simulink model "doublMassControl"  (R2016b)
settings: Solver=VariableStepAuto  StartTime=0.0  StopTime=0.4  FixedStep=2e-4  RelTol=1e-3
values from neighbouring files (symbols this model uses):
  denGp = [m1*m2 0 (m1+m2)*k 0 0]    [doubleMassInit.m]
  denominator = denominator{1}    [doubleMassInit.m]    (also in mainFeedbackTuning.m)
  denQ = [1 2*wq*0.707 wq*wq]    [doubleMassInit.m]
  fs = 5000*2    (= 10000)    [doubleMassInit.m]    (also in mainFeedbackTuning.m)
  k = wn*wn*m1*m2/(m1+m2)    (= 25266187.2668)    [doubleMassInit.m]
  m11 = m1-1    (= 19)    [doubleMassInit.m]
  m22 = m2-0.5    (= 4.5)    [doubleMassInit.m]
  numerator = numerator{1}    [doubleMassInit.m]    (also in mainFeedbackTuning.m)
  numGp = k    (= 25266187.2668)    [doubleMassInit.m]
  numQ = wq*wq    (= 1421223033.76)    [doubleMassInit.m]
  Ts = 1/fs    (= 0.0001)    [doubleMassInit.m]    (also in mainFeedbackTuning.m)
libraries: simulink x6, model_controller x1
settings Model: Creator=Dai Luyao  LastModifiedBy=Dai Luyao

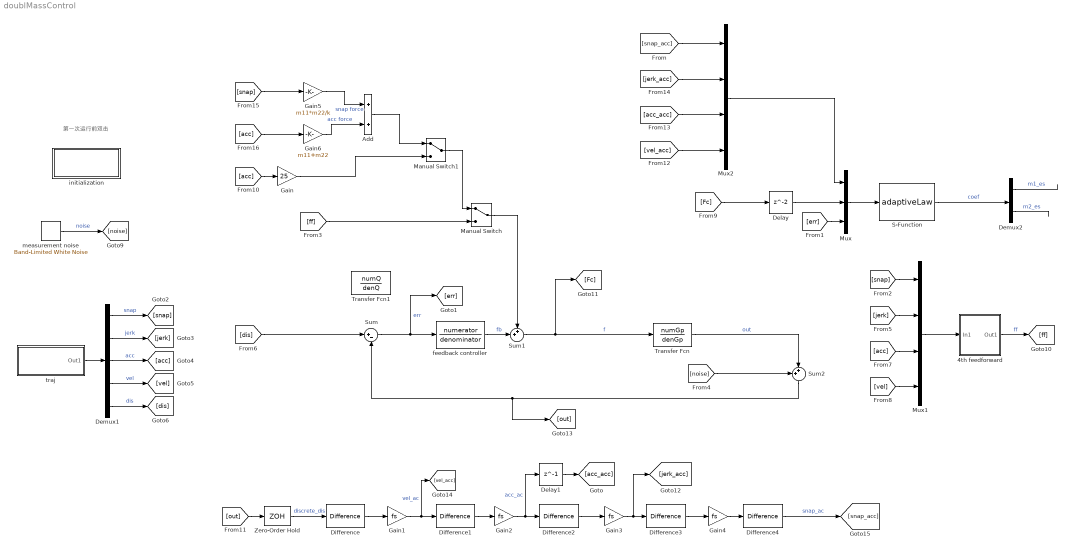
== system doublMassControl ==
  note: 第一次运行前双击
  4th feedforward : Subsystem
  Add : Sum
  Delay : Delay
  Delay1 : Delay  DelayLength=1
  Demux1 : Demux  Outputs=5
  Demux2 : Demux  Outputs=2
  Difference{,1..4} (5 alike) : simulink/Discrete/Difference  ICPrevInput=0.0  OutMin=[]  OutMax=[]  OutDataType=fixdt(1, 16)  OutScaling=2^-10  DoSatur=off
  Gain : Gain  Gain=25
  Gain{1..4} (4 alike) : Gain  Gain=fs
  Gain5 : Gain  Gain=m11*m22/k
  Gain6 : Gain  Gain=m11+m22
  Manual Switch : ManualSwitch
  Manual Switch1 : ManualSwitch
  Mux : Mux  Inputs=3
  Mux1 : Mux
  Mux2 : Mux
  S-Function : S-Function  FunctionName=adaptiveLaw  Parameters=1  SFunctionDeploymentMode=off  EnableBusSupport=off
  Sum : Sum  Inputs=|+-
  Sum1 : Sum  Inputs=++|
  Sum2 : Sum  Inputs=++|
  Transfer Fcn : TransferFcn  Numerator=numGp  Denominator=denGp
  Transfer Fcn1 : TransferFcn  Numerator=numQ  Denominator=denQ
  Zero-Order Hold : ZeroOrderHold  SampleTime=Ts
  feedback controller : TransferFcn  Numerator=numerator  Denominator=denominator
  initialization : Subsystem
      settings: OpenFcn=doubleMassInit;  MoveFcn=edit doubleMassInit;
  measurement noise : simulink/Sources/Band-Limited White Noise  Cov=noisePower  Ts=Ts  seed=[23341]
  traj : Subsystem  BlockChoice=4th order traj
      settings: AttributesFormatString=%<BlockChoice>  TemplateBlock=model_controller/Profile Generators/traj  MemberBlocks=2th order traj,3rd order traj,4th order traj,step
  wires:
  Sum/1 -> feedback controller/1, [err]  "err"
  feedback controller/1 -> Sum1/2  "fb"
  Sum1/1 -> Transfer Fcn/1, [Fc]  "f"
  Difference1/1 -> Gain2/1
  Difference/1 -> Gain1/1
  Gain1/1 -> [vel_acc], Difference1/1  "vel_ac"
  Mux/1 -> S-Function/1
  S-Function/1 -> Demux2/1  "coef"
  Zero-Order Hold/1 -> Difference/1  "discrete_dis"
  [err] -> Mux/3
  Delay/1 -> Mux/2
  Mux1/1 -> 4th feedforward/1(In1)
  measurement noise/1 -> [noise]  "noise"
  Transfer Fcn/1 -> Sum2/2  "out"
  [noise] -> Sum2/1
  Sum2/1 -> [out], Sum/2
  Demux1/1 -> [snap]  "snap"
  Demux1/2 -> [jerk]  "jerk"
  Demux1/3 -> [acc]  "acc"
  Demux1/4 -> [vel]  "vel"
  Demux1/5 -> [dis]  "dis"
  traj/1(Out1) -> Demux1/1
  [vel] -> Mux1/4
  [acc] -> Mux1/3
  [jerk] -> Mux1/2
  [snap] -> Mux1/1
  4th feedforward/1(Out1) -> [ff]  "ff"
  [Fc] -> Delay/1
  Difference2/1 -> Gain3/1
  Gain2/1 -> Delay1/1, Difference2/1  "acc_ac"
  Gain3/1 -> [jerk_acc], Difference3/1
  Gain4/1 -> Difference4/1
  Difference3/1 -> Gain4/1
  [out] -> Zero-Order Hold/1
  Difference4/1 -> [snap_acc]  "snap_ac"
  [snap_acc] -> Mux2/1
  [jerk_acc] -> Mux2/2
  [acc_acc] -> Mux2/3
  [vel_acc] -> Mux2/4
  Mux2/1 -> Mux/1
  Delay1/1 -> [acc_acc]
  Demux2/1 -> ?  "m1_es"
  Demux2/2 -> ?  "m2_es"
  [acc] -> Gain/1
  [snap] -> Gain5/1
  [acc] -> Gain6/1
  Gain5/1 -> Add/1  "snap force"
  Gain6/1 -> Add/2  "acc force"
  Add/1 -> Manual Switch1/1
  Gain/1 -> Manual Switch1/2
  Manual Switch1/1 -> Manual Switch/1
  [dis] -> Sum/1
  [ff] -> Manual Switch/2
  Manual Switch/1 -> Sum1/1

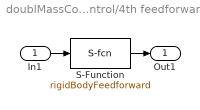
== system doublMassControl/4th feedforward ==
  In1 : Inport
  S-Function : S-Function  FunctionName=rigidBodyFeedforward  SFunctionDeploymentMode=off  EnableBusSupport=off
  Out1 : Outport
  wires:
  In1/1 -> S-Function/1
  S-Function/1 -> Out1/1

== system doublMassControl/initialization ==

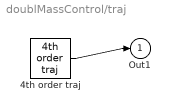
== system doublMassControl/traj ==
  4th order traj : model_controller/Profile Generators/4th order traj  t0=0  x=0.06  v=0.25  a=10  j=800  d=64000  Ts=0
  Out1 : Outport
  wires:
  4th order traj/1 -> Out1/1
